simulink model "BRS_Tay"  (R2017b)
settings: Solver=FixedStepDiscrete  StartTime=0.0  StopTime=1.0  FixedStep=1.0  RelTol=1e-3  EnableMultiTasking=on
libraries: taXlibrary x8
settings Model: Creator=emmert  LastModifiedBy=shuai
settings DataIOCC: LimitDataPoints=on  SaveFormat=Array  SignalLoggingSaveFormat=ModelDataLogs
settings OptimizationCC: ExpressionDepthLimit=2147483647  LifeSpan=inf
settings DebuggingCC: UnderspecifiedInitializationDetection=Classic  MergeDetectMultiDrivingBlocksExec=none  SolverPrmCheckMsg=warning  FcnCallInpInsideContextMsg=warning  StateNameClashWarn=warning  SFUnexpectedBacktrackingDiag=warning  SFNoUnconditionalDefaultTransitionDiag=warning  SFExecutionAtInitializationDiag=none
settings HardwareCC: ProdBitPerPointer=32  ProdBitPerSizeT=32  ProdBitPerPtrDiffT=32  ProdLargestAtomicFloat=None  ProdIntDivRoundTo=Undefined  ProdEndianess=Unspecified  ProdWordSize=32  ProdHWDeviceType=32-bit Generic
settings ModelReferenceCC: PropagateSignalLabelsOutOfModel=off
settings CodeAppCC: StateflowObjectComments=on
settings GRTTargetCC: TargetLangStandard=C89/C90 (ANSI)  GeneratePreprocessorConditionals=Disable all  CombineOutputUpdateFcns=off  GRTInterface=on
settings ConfigComp: CovMetricSettings=dw  CovHtmlReporting=on  CovSaveCumulativeToWorkspaceVar=on  CovSaveSingleToWorkspaceVar=on  CovExternalEMLEnable=off  CovSFcnEnable=off

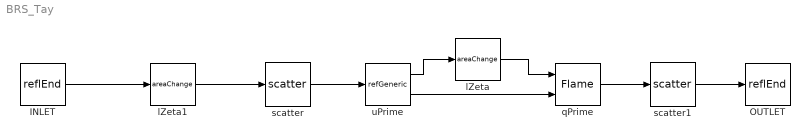
== system BRS_Tay ==
  INLET : taXlibrary/reflEnd  element=reflEnd  loc=Upstream  r=0  A=0.031416  Mach=11.3*0.001056/0.031416/sqrt(1.4*287.04*293)  rho=101325/(287.04*293)  c=sqrt(1.4*287.04*293)
      settings: AttributesFormatString=%<r>
  OUTLET : taXlibrary/reflEnd  element=reflEnd  loc=Downstream  r=0  A=[]  Mach=[]  rho=[]  c=[]
      settings: AttributesFormatString=%<r>
  lZeta : taXlibrary/areaChange  element=lZeta  zeta=0  lred=0  leff=0  l=1  A=90*90/1000^2
  lZeta1 : taXlibrary/areaChange  element=lZeta  zeta=1  lred=0  leff=0  l=1  A=pi/4*((40/1000)^2-(16/1000)^2)
  qPrime : taXlibrary/Flame  element=rankineHugoniot  nRef=1  Mach=0.001056*101325/(287.04*293)*11.3/(101325/(287.04*1930)*0.0081*sqrt(1.4*287.04*1930))  rho=101325/(287.04*1930)  c=sqrt(1.4*287.04*1930)
  scatter : taXlibrary/scatter  element=scatteringDummy  loc=Upstream
  scatter1 : taXlibrary/scatter  element=scatteringDummy  loc=Downstream
  uPrime : taXlibrary/refGeneric  element=reference  filename=model4tax.mat  modelname=model4tax  active=off
      settings: AttributesFormatString=%<modelname>
  wires:
  lZeta/1 -> qPrime/1
  qPrime/1 -> scatter1/1
  uPrime/1 -> lZeta/1
  uPrime/2 -> qPrime/2
  scatter1/1 -> OUTLET/1
  lZeta1/1 -> scatter/1
  scatter/1 -> uPrime/1
  INLET/1 -> lZeta1/1
